simulink model "Test_Freq_Resp_1"  (Simulink 8.3)
settings: Solver=ode4  StartTime=0.0  StopTime=N-1  FixedStep=T  RelTol=1e-3
undefined symbols (not defined in the file): A, N, T, w_end, w_start
settings Model: Creator=baqumau  LastModifiedBy=baqumau
settings DataIOCC: SignalLoggingSaveFormat=Dataset
settings DebuggingCC: UnderspecifiedInitializationDetection=Simplified  StateNameClashWarn=none
settings GRTTargetCC: CombineOutputUpdateFcns=on  GRTInterface=off

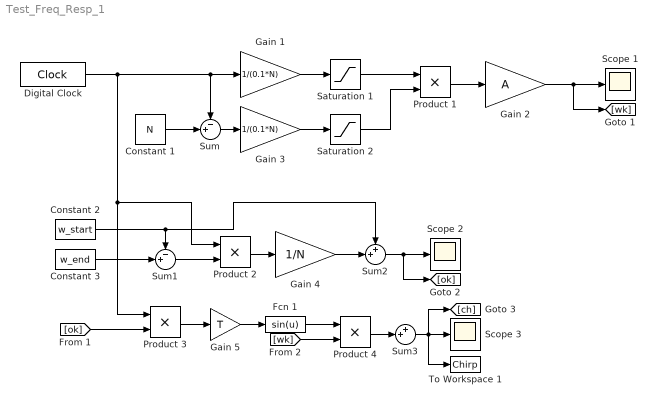
== system Test_Freq_Resp_1 ==
  Constant 1 : Constant  Value=N
  Constant 2 : Constant  Value=w_start
  Constant 3 : Constant  Value=w_end
  Digital Clock : DigitalClock  SampleTime=T
  Fcn 1 : Fcn  Expr=sin(u)
  Gain 1 : Gain  Gain=1/(0.1*N)
  Gain 2 : Gain  Gain=A
  Gain 3 : Gain  Gain=1/(0.1*N)
  Gain 4 : Gain  Gain=1/N
  Gain 5 : Gain  Gain=T
  Product {1..4} (4 alike) : Product
  Saturation 1 : Saturate  UpperLimit=1  LowerLimit=-1
  Saturation 2 : Saturate  UpperLimit=1  LowerLimit=-1
  Scope 1 : Scope
  Scope 2 : Scope
  Scope 3 : Scope
      settings: SaveName=ScopeData2
  Sum : Sum  Inputs=-+|
  Sum1 : Sum  Inputs=-+|
  Sum2 : Sum  Inputs=++|
  Sum3 : Sum  Inputs=++|
  To Workspace 1 : ToWorkspace  VariableName=Chirp  SaveFormat=Structure With Time  SampleTime=-1
  wires:
  Gain 1/1 -> Saturation 1/1
  Saturation 1/1 -> Product 1/1
  Digital Clock/1 -> Product 3/1, Product 2/1, Gain 1/1, Sum/1
  Sum/1 -> Gain 3/1
  Constant 1/1 -> Sum/2
  Gain 3/1 -> Saturation 2/1
  Saturation 2/1 -> Product 1/2
  Product 1/1 -> Gain 2/1
  Gain 2/1 -> [wk], Scope 1/1
  Constant 2/1 -> Sum2/1, Sum1/1
  Constant 3/1 -> Sum1/2
  Sum1/1 -> Product 2/2
  Product 2/1 -> Gain 4/1
  Gain 4/1 -> Sum2/2
  Sum2/1 -> [ok], Scope 2/1
  [ok] -> Product 3/2
  Product 3/1 -> Gain 5/1
  Gain 5/1 -> Fcn 1/1
  Fcn 1/1 -> Product 4/1
  [wk] -> Product 4/2
  Product 4/1 -> Sum3/2
  Sum3/1 -> [ch], To Workspace 1/1, Scope 3/1
